simulink model "SiMappedEngineV"  (R2018a)
settings: Solver=FixedStepAuto  StartTime=0.0  StopTime=inf  FixedStep=0.001  RelTol=1e-3  EnableMultiTasking=on
model workspace (MAT data in the model file):
  Cps = 2
  F0z = [6086.4 4324.8]
  F_reff = 0.07394
  F_zmax = 10000
  F_zmin = 100
  F_zo = 4000
  Kz = 48000
  MF.f.mu_x = 1.2
  MF.f.mu_y = 0.935
  MF.f.Bx = 11.7
  MF.f.By = 8.86
  MF.f.Cx = 1.69
  MF.f.Cy = 1.19
  MF.f.Ex = 0.377
  MF.f.Ey = -1.21
  MF.f.Cxalpha = 1.09
  MF.f.Cykappa = 1.08
  MF.f.Bx1 = 12.4
  MF.f.Bx2 = -10.8
  MF.f.By1 = 6.46
  MF.f.By2 = 4.2
  MF.f.Sh = 0
  MF.f.Sv = 0
  MF.r.mu_x = 1.2
  MF.r.mu_y = 0.961
  MF.r.Bx = 11.1
  MF.r.By = 9.3
  MF.r.Cx = 1.69
  MF.r.Cy = 1.19
  MF.r.Ex = 0.362
  MF.r.Ey = -1.11
  MF.r.Cxalpha = 1.09
  MF.r.Cykappa = 1.08
  MF.r.Bx1 = 12.4
  MF.r.Bx2 = -10.8
  MF.r.By1 = 6.46
  MF.r.By2 = 4.2
  MF.r.Sh = 0
  MF.r.Sv = 0
  NCyl = 6
  NE_VEC = [800 1200 1600 2000 2400 2800 3200 3600 4000 4400 4800]
  Pstd = 101325
  Rair = 287
  Tstd = 293.15
  Vd = 0.00346
  f_air = [0 0 0 0 0 0 0 0 0 0 0 0 ... (256 elements, 16x16)]
  f_co = [0 0 0 0 0 0 0 0 0 0 0 0 ... (256 elements, 16x16)]
  f_co2 = [0 0 0 0 0 0 0 0 0 0 0 0 ... (256 elements, 16x16)]
  f_eff = [352.135682859 352.135682859 320.724378192 303.655312657 295.930136708 291.240087194 291.240271258 291.240312459 291.240275452 291.240198499 291.240100781 291.240018769 ... (256 elements, 16x16)]
  f_fuel = [0 0 0 0 0 0 0 0 0 0 0 0 ... (256 elements, 16x16)]
  f_hc = [0 0 0 0 0 0 0 0 0 0 0 0 ... (256 elements, 16x16)]
  f_nox = [0 0 0 0 0 0 0 0 0 0 0 0 ... (256 elements, 16x16)]
  f_pm = [0  0  0  0  0  0  0  0  0  0  0  0  0  0  0  0; 0  0  0  0  0  0  0  0  0  0  0  0  0  0  0  0; 0  0  0  0  0  0  0  0  0  0  0  0  0  0  0  0; 0  0  0  0  0  0  0  0  0  0  0  0  0  0  0  0; 0  0  0  0  0  0  0  0  0  0  0  0  0  0  0  0; 0  0  0  0  0  0  0  0  0  0  0  0  0  0  0  0; 0  0  0  0  0  0  0  0  0  0  0  0  0  0  0  0; 0  0  0  0  0  0  0  0  0  0  0  0  0  0  0  0; 0  0  0  0  0  0  0  0  0  0  0  0  0  0  0  0; 0  0  0  0  0  0  0  0  0  0  0  0  0  0  0  0; 0  0  0  0  0  0  0  0  0  0  0  0  0  0  0  0; 0  0  0  0  0  0  0  0  0  0  0  0  0  0  0  0; 0  0  0  0  0  0  0  0  0  0  0  0  0  0  0  0; 0  0  0  0  0  0  0  0  0  0  0  0  0  0  0  0; 0  0  0  0  0  0  0  0  0  0  0  0  0  0  0  0; 0  0  0  0  0  0  0  0  0  0  0  0  0  0  0  0]
  f_susp_axl_bp = [1 2]
  f_susp_dz_bp = [-4 -0.14 -0.13 -0.12 -0.11 -0.1 -0.09 -0.08 -0.07 -0.06 -0.05 -0.04 -0.03 -0.02 -0.01 0 0.01 0.02 0.03 0.04 0.05 0.06 0.07 0.08 0.09 0.1 0.11 0.12 0.13 0.14 4]
  f_susp_dzdot_bp = [-4 -0.14 -0.13 -0.12 -0.11 -0.1 -0.09 -0.08 -0.07 -0.06 -0.05 -0.04 -0.03 -0.02 -0.01 0 0.01 0.02 0.03 0.04 0.05 0.06 0.07 0.08 0.09 0.1 0.11 0.12 0.13 0.14 4]
  f_susp_fmz = [-213379.591456 -28099.591456 -27619.591456 -27139.591456 -26659.591456 -26179.591456 -25699.591456 -25219.591456 -24739.591456 -24259.591456 -23779.591456 -23299.591456 ... (468968 elements, 31x31x61x2x4)]
  f_susp_geom = [-0.832564012244 0.043269987756 0.045538987756 0.047807987756 0.050076987756 0.052345987756 0.054614987756 0.056883987756 0.059152987756 0.061421987756 0.063690987756 0.065959987756 ... (11346 elements, 31x61x2x3)]
  f_susp_strgdelta_bp = [-0.523598775598 -0.506145483078 -0.488692190558 -0.471238898038 -0.453785605519 -0.436332312999 -0.418879020479 -0.401425727959 -0.383972435439 -0.366519142919 -0.349065850399 -0.331612557879 -0.314159265359 -0.296705972839 -0.279252680319 -0.261799387799 -0.244346095279 -0.226892802759 -0.209439510239 -0.191986217719 -0.174532925199 -0.157079632679 -0.13962634016 -0.12217304764 -0.10471975512 -0.0872664625997 -0.0698131700798 -0.0523598775598 -0.0349065850399 -0.0174532925199 0 0.0174532925199 0.0349065850399 0.0523598775598 0.0698131700798 0.0872664625997 0.10471975512 0.12217304764 0.13962634016 0.157079632679 0.174532925199 0.191986217719 0.209439510239 0.226892802759 0.244346095279 0.261799387799 0.279252680319 0.296705972839 0.314159265359 0.331612557879 0.349065850399 0.366519142919 0.383972435439 0.401425727959 0.418879020479 0.436332312999 0.453785605519 0.471238898038 0.488692190558 0.506145483078 0.523598775598]
  f_tbrake = [0 76.8593923996 105.140482948 131.533638111 157.926793274 176.658631717 176.65727296 176.656856686 176.656879077 176.657093756 176.657404516 176.65772406 ... (256 elements, 16x16)]
  f_tbrake_n_bpt = [0 649.519052838 912.419621844 1175.32019085 1438.22075986 1701.12132886 1964.02189787 2226.92246687 2489.82303588 2752.72360489 3015.62417389 3278.5247429 3541.4253119 3804.32588091 4067.22644992 4330.12701892]
  f_tbrake_t_bpt = [0 34.6410161514 61.0341713143 87.4273264773 113.82048164 140.213636803 166.606791966 192.999947129 219.393102292 245.786257455 272.179412618 298.572567781 324.965722944 351.358878107 377.75203327 404.145188433]
  f_texh = [766.752464599 766.752464599 786.17542386 801.679939032 884.591982581 910.574397722 910.571871054 910.570774534 910.570601632 910.570821151 910.571247242 910.571639815 ... (256 elements, 16x16)]
  f_twc_eff_co = [0.17 0.25 0.45 0.99 0.99 0.99 0.99]
  f_twc_eff_hc = [0.21 0.375 0.75 0.98 0.98 0.98 0.98]
  f_twc_eff_lam = [0.909090909 0.944055944 0.979020979 1 1.013986014 1.048951049 1.083916084]
  f_twc_eff_nox = [0.98 0.98 0.98 0.97 0.05 0.02 0]
  h = 0.5
  k_z = 50
  kappa_max = 1.5
  kappa_min = -1.5
  lam_Cx = 1
  lam_Cy = 1
  lam_Cz = 1
  lam_Ex = 1
  lam_Ey = 1
  lam_F_zo = 1
  lam_Hx = 1
  lam_Hy = 1
  lam_Kxkappa = 1
  lam_Kyalpha = 1
  lam_Kygamma = 1
  lam_Kzgamma = 1
  lam_Mr = 1
  lam_Mx = 1
  lam_My = 1
  lam_S = 1
  lam_VMx = 1
  lam_Vx = 1
  lam_Vy = 1
  lam_Vykappa = 1
  lam_muV = 0
  lam_mux = 1
  lam_muy = 1
  lam_t = 1
  lam_xalpha = 1
  lam_ykappa = 1
  numWheel = 4
  p_Cx1 = 1.579
  p_Cy1 = 1.3332
  p_Dx1 = 1.0422
  p_Dx2 = -0.08285
  p_Dx3 = 0
  p_Dy1 = 0.8784
  p_Dy2 = -0.06445
  p_Dy3 = 0
  p_Ex1 = 0.11185
  p_Ex2 = 0.3127
  p_Ex3 = 0
  p_Ex4 = 0.001603
  p_Ey1 = -0.8227
  p_Ey2 = -0.6062
  p_Ey3 = 0.09825
  p_Ey4 = -6.546
  p_Ey5 = 0
  p_Fz1 = 0.7098
  p_Hx1 = 0.00021585
  p_Hx2 = 0.0011538
  p_Hy1 = -0.0018043
  p_Hy2 = 0.003518
  p_Kx1 = 21.69
  p_Kx2 = 13.774
  p_Kx3 = -0.4119
  p_Ky1 = -15.314
  p_Ky2 = 1.7044
  p_Ky3 = 0.36986
  p_Ky4 = 1.9896
  p_Ky5 = 0
  p_Ky6 = -0.9004
  p_Ky7 = -0.2328
  p_Vx1 = 1.5973e-05
  p_Vx2 = 0.0001043
  p_Vy1 = -0.006642
  p_Vy2 = 0.03597
  p_Vy3 = -0.1621
  p_Vy4 = -0.4908
  p_pmx1 = 0
  p_px1 = -0.3489
  p_px2 = 0.382
  p_px3 = -0.09634
  p_px4 = 0.06447
  p_py1 = -0.6249
  p_py2 = -0.06535
  p_py3 = -0.1668
  p_py4 = 0.2834
  p_py5 = 0
libraries: autolibutils x2, autolibsharedmappedengines x1
settings Model: ModifiedByFormat=The MathWorks, Inc.  Creator=The MathWorks, Inc.  LastModifiedBy=The MathWorks, Inc.
settings SolverCC: DecoupledContinuousIntegration=on
settings DataIOCC: DSMLogging=off
settings CodeAppCC: StateflowObjectComments=on
settings GRTTargetCC: TargetLangStandard=C89/C90 (ANSI)
settings ConfigComp: CovMetricSettings=dsw  CovHtmlReporting=on  CovSaveCumulativeToWorkspaceVar=on  CovSaveSingleToWorkspaceVar=on  CovShowResultsExplorer=off  CovExternalEMLEnable=off
settings SimscapeCC: SimscapeNormalizeSystem=off  SimscapeNominalValues={1, 'bar'; 1, 'cm^3/s'; 1, 'bar*kg/s'; 1, 'kJ/kg'; 1, 'kW'}

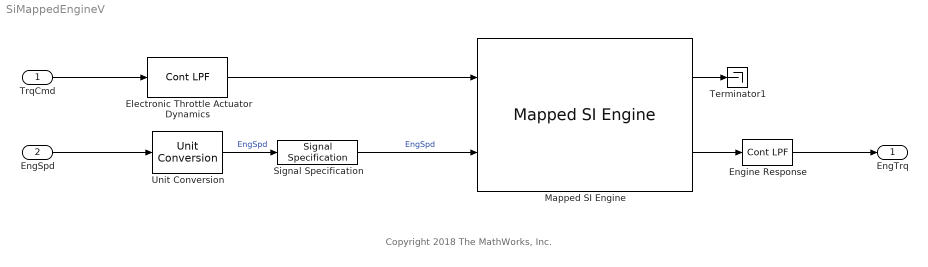
== system SiMappedEngineV ==
  note: Copyright 2018 The MathWorks, Inc.
  TrqCmd : Inport
  EngSpd : Inport  Port=2  Unit=rad/s
  Electronic Throttle Actuator Dynamics : autolibutils/Cont LPF  wc=2*pi/.085  aMode=2
      settings: SourceProductName=Powertrain Blockset  SourceProductBaseCode=PW
  Engine Response : autolibutils/Cont LPF  wc=40*2*pi  aMode=2
      settings: SourceProductName=Powertrain Blockset  SourceProductBaseCode=PW
  Mapped SI Engine : autolibsharedmappedengines/Mapped SI Engine  TurboLagCheckbox=off  rowVarName=TrqCmd  f_tbrake_t_bpt=f_tbrake_t_bpt  colVarName=EngSpd  f_tbrake_n_bpt=f_tbrake_n_bpt  NCyl=NCyl  Cps=Cps  Vd=Vd  Rair=Rair  Pstd=Pstd  Tstd=Tstd  Use1=on  Use2=on  Use3=on  Use4=on  Use5=on  Use6=on  Use7=on  Use8=on  Use9=on  Use10=off  f_tbrake_bst=[0, 79.51 81.38 91.45 97.78 102.6 106.2 109.6 111.6 113.4 113.9 113.3 115 111.9 108.1 105]  tau_thr=0.2  tau_bst_rising=1.5  tau_bst_falling=1  tq_blend_frac=0.01  Name1=Brake Torque  f_tbrake=f_tbrake  Name2=Air Mass Flow  f_air=f_air  Name3=Fuel Flow  f_fuel=f_fuel  Name4=Exhaust Temperature  f_texh=f_texh  Name5=[514.035834811904 472.420001567292 468.560027988283 467.25113080026 469.376552017678 472.466817198703 477.085817372135 482.089315297269 488.091390331625 495.511698221518 503.603605470575 513.545560314063 524.708632042863 537.901582788691 547.57773149968;372.215126833557 362.023004934345 357.061196096605 354.397690627091 353.695017513094 355.069365264177 357.083429546077 359.150328797338 361.216056662124 363.787443052002 368.052362907894 373.273609540704 379.492527390704 387.062712835118 392.829054841793;326.61409907784 316.864439849348 311.950172215081 309.623392513349 308.520317680707 308.639621388036 309.473192508284 311.206605049837 312.435624355117 314.372691523229 315.240918825382 319.20290576235 323.194337587902 328.582300779183 332.542719046893;302.302708332089 292.988583490457 288.191388571794 286.11397076702 285.309041994516 284.733243126823 284.189019193475 282.574319206257 284.12037910983 287.79556805798 288.17907837576 290.209859138972 293.679673638155 297.45343144841 300.726288347892;288.700928736811 278.551672830084 273.400833959319 270.536547804349 267.833435583205 267.119414364878 265.972950018046 266.740920363958 268.048224971445 270.838385340352 270.778373480454 272.970259132319 275.506872347887 278.72040783414 281.813869092965;284.845821006168 269.394829178651 263.982926589081 260.478586413209 257.028965789929 255.931084916756 255.874470882376 256.430426703396 258.42024291946 257.808327020541 258.950655075076 261.079050323518 263.461085730423 266.38231289239 269.295763051135;288.386442360439 264.344752526028 257.213462364171 254.168296127581 250.527881300837 249.049345022729 250.073316495023 249.665324624047 248.602086912424 249.355944667699 250.714426186754 252.515083416491 254.990022645247 258.139224389126 258.88586921331;288.386442360439 267.197275532715 251.193959608514 247.553061326459 246.301141111655 244.695607301207 242.621990784403 242.304630618562 242.866111727694 243.758994026591 244.970247326866 246.821991594926 249.775586923996 251.245282116681 253.478417008787;288.386442360439 277.668290802935 252.854894387889 243.851167532952 241.861572413297 238.689990387976 238.067198500515 238.072941982365 238.685701547209 239.312989651019 240.673403883432 242.669277941474 245.301951037108 246.789302536782 247.789414843363;288.386442360439 277.504945286633 270.702819258252 245.731480615597 238.395305310031 236.119281963407 235.324944828075 235.181758472016 235.88354482046 236.67974458838 237.758701429304 239.923633193373 242.123394230695 242.998011528535 244.273734537053;288.386442360439 277.504945286633 279.349376222353 263.18046263446 241.569205761561 235.781254475789 234.445285156959 234.881842747232 234.822376790859 235.79445272942 237.439515459863 239.43946089678 241.356663529347 242.334213324245 244.486434215002;288.386442360439 277.504945286633 279.349376222353 299.505188255346 260.338046997911 239.40420517855 235.256510952508 234.880694514868 234.31593804329 236.319225658558 237.102712721133 239.012709272806 240.75776355138 241.336977805019 256.331160738088;288.386442360439 277.504945286633 279.349376222353 299.505188255346 320.026630425816 342.9283130372 241.52452305243 328.315966517739 244.549289572305 251.858270967766 240.732881082116 242.07382019702 244.535478307747 249.496579565711 263.930188372987;288.386442360439 277.504945286633 279.349376222353 299.505188255346 320.026630425816 342.9283130372 345.883623776508 328.315966517739 317.337354078743 314.624789096503 254.725548546873 250.384805432702 271.371327381584 265.474840242786 277.521724347837;288.386442360439 277.504945286633 279.349376222353 299.505188255346 320.026630425816 342.9283130372 345.883623776508 328.315966517739 319.749039003082 318.879022253509 311.782458169383 312.350604651759 319.747883103035 320.841917879101 308.256263223954]  f_eff=f_eff  Name6=EO HC  f_hc=f_hc  Name7=EO CO  f_co=f_co  Name8=EO NOx  f_nox=f_nox  Name9=EO CO2  f_co2=f_co2  Name10=Brake Torque  f_pm=f_pm  aMode=2
      settings: SourceProductName=Powertrain Blockset  SourceProductBaseCode=PW
  Signal Specification : SignalSpecification  Unit=rpm
  Terminator1 : Terminator
  Unit Conversion : UnitConversion
  EngTrq : Outport
  wires:
  Mapped SI Engine/2 -> Engine Response/1
  Unit Conversion/1 -> Signal Specification/1  "EngSpd"
  TrqCmd/1 -> Electronic Throttle Actuator Dynamics/1
  Electronic Throttle Actuator Dynamics/1 -> Mapped SI Engine/1
  Signal Specification/1 -> Mapped SI Engine/2  "EngSpd"
  EngSpd/1 -> Unit Conversion/1
  Mapped SI Engine/1 -> Terminator1/1
  Engine Response/1 -> EngTrq/1
